simulink model "LPV_TorqueTracker_DT_CP_LMI_II_v3"  (R2018a)
settings: Solver=VariableStepAuto  StartTime=0  StopTime=FA.TMax  FixedStep=Simulation.DT  RelTol=1e-3  EnableMultiTasking=on
undefined symbols (not defined in the file or in its folder): Control, DiscIntNeverNeededParam, FA, OutList, Parameters, PitchControlParams, rpm2radps, strmatch, TorqueControlParams
libraries: simulink_extras x1
settings Model: ExtModeTrigMode=oneshot  ExtModeArmWhenConnect=off  Creator=Dana Martin  LastModifiedBy=dmartin
settings DataIOCC: SaveFormat=Array  SaveOutput=off  InspectSignalLogs=on  SignalLoggingName=sigsOut  OutputTimes=[0:500]/50
settings OptimizationCC: BooleanDataType=off  ExpressionDepthLimit=2147483647  InitFltsAndDblsToZero=on  LifeSpan=inf
settings DebuggingCC: SignalRangeChecking=warning  SaveWithParameterizedLinksMsg=none  UnderspecifiedInitializationDetection=Classic  MergeDetectMultiDrivingBlocksExec=none  SignalResolutionControl=TryResolveAllWithWarning  TimeAdjustmentMsg=warning  MultiTaskDSMMsg=warning  MultiTaskCondExecSysMsg=warning  ParameterUnderflowMsg=warning  UnderSpecifiedDataTypeMsg=warning  UnnecessaryDatatypeConvMsg=warning  VectorMatrixConversionMsg=warning  FcnCallInpInsideContextMsg=warning  SignalLabelMismatchMsg=warning  SFcnCompatibilityMsg=warning  UniqueDataStoreMsg=warning  AllowSymbolicDim=off  ModelReferenceIOMsg=warning  ModelReferenceVersionMismatchMessage=warning  ModelReferenceIOMismatchMessage=warning  StateNameClashWarn=warning  StrictBusMsg=WarnOnBusTreatedAsVector  NonBusSignalsTreatedAsBus=warning  SFUnexpectedBacktrackingDiag=warning  SFNoUnconditionalDefaultTransitionDiag=warning  SFExecutionAtInitializationDiag=none
settings HardwareCC: ProdBitPerPointer=32  ProdBitPerSizeT=32  ProdBitPerPtrDiffT=32  ProdLargestAtomicFloat=None  ProdIntDivRoundTo=Undefined  ProdEndianess=Unspecified  ProdWordSize=32  ProdHWDeviceType=32-bit Generic  TargetBitPerPointer=64  TargetBitPerSizeT=64  TargetBitPerPtrDiffT=64  TargetLongLongMode=on  TargetIntDivRoundTo=Zero  TargetEndianess=LittleEndian  TargetWordSize=64  TargetHWDeviceType=MATLAB Host  ProdEqTarget=off
settings ModelReferenceCC: PropagateSignalLabelsOutOfModel=off
settings CodeAppCC: StateflowObjectComments=on
settings GRTTargetCC: TargetFcnLib=ansi_tfl_tmw.mat  TargetLangStandard=C89/C90 (ANSI)  ModelReferenceCompliant=off  GeneratePreprocessorConditionals=Disable all  CombineOutputUpdateFcns=off  GRTInterface=on
settings ConfigComp: CovMetricSettings=dw  CovHtmlReporting=on  CovSaveCumulativeToWorkspaceVar=on  CovSaveSingleToWorkspaceVar=on  CovExternalEMLEnable=off  CovSFcnEnable=off

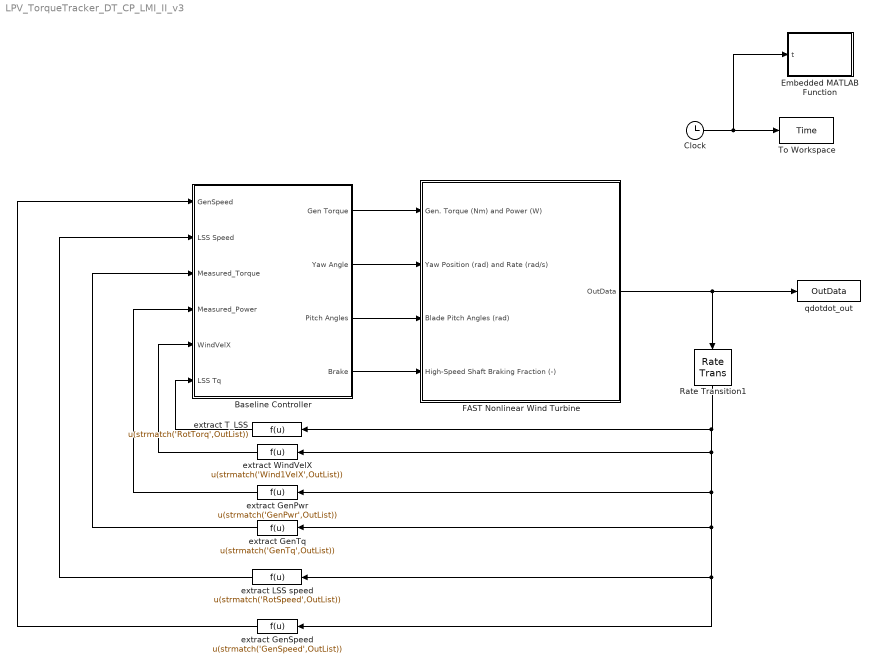
== system LPV_TorqueTracker_DT_CP_LMI_II_v3 ==
  Baseline Controller : Subsystem
  Clock : Clock
  Embedded MATLAB Function : MATLAB Function  TreatAsAtomicUnit=on
  FAST Nonlinear Wind Turbine : Subsystem  mask(FAST Nonlinear Wind Turbine){}
      mask help: This block contains the FAST S-Function.
      mask init:
      | clear FAST_SFunc
  Rate Transition1 : RateTransition
  To Workspace : ToWorkspace  VariableName=Time  SampleTime=FA.DT
  extract GenPwr : Fcn  Expr=u(strmatch('GenPwr',OutList))
  extract GenSpeed : Fcn  Expr=u(strmatch('GenSpeed',OutList))
  extract GenTq : Fcn  Expr=u(strmatch('GenTq',OutList))
  extract LSS speed : Fcn  Expr=u(strmatch('RotSpeed',OutList))
  extract T_LSS : Fcn  Expr=u(strmatch('RotTorq',OutList))
  extract WindVelX : Fcn  Expr=u(strmatch('Wind1VelX',OutList))
  qdotdot_out : ToWorkspace  VariableName=OutData  SaveFormat=Structure With Time  SampleTime=-1
  wires:
  Clock/1 -> Embedded MATLAB Function/1(t), To Workspace/1
  Baseline Controller/1(Gen Torque) -> FAST Nonlinear Wind Turbine/1(Gen. Torque (Nm) and Power (W))
  Baseline Controller/3(Pitch Angles) -> FAST Nonlinear Wind Turbine/3(Blade Pitch Angles (rad))
  extract GenSpeed/1 -> Baseline Controller/1(GenSpeed)
  Baseline Controller/2(Yaw Angle) -> FAST Nonlinear Wind Turbine/2(Yaw Position (rad) and Rate (rad/s))
  Baseline Controller/4(Brake) -> FAST Nonlinear Wind Turbine/4(High-Speed Shaft Braking Fraction (-))
  extract LSS speed/1 -> Baseline Controller/2(LSS Speed)
  extract GenPwr/1 -> Baseline Controller/4(Measured_Power)
  FAST Nonlinear Wind Turbine/1(OutData) -> qdotdot_out/1, Rate Transition1/1
  extract GenTq/1 -> Baseline Controller/3(Measured_Torque)
  extract WindVelX/1 -> Baseline Controller/5(WindVelX)
  extract T_LSS/1 -> Baseline Controller/6(LSS Tq)
  Rate Transition1/1 -> extract T_LSS/1, extract WindVelX/1, extract LSS speed/1, extract GenSpeed/1, extract GenTq/1, extract GenPwr/1

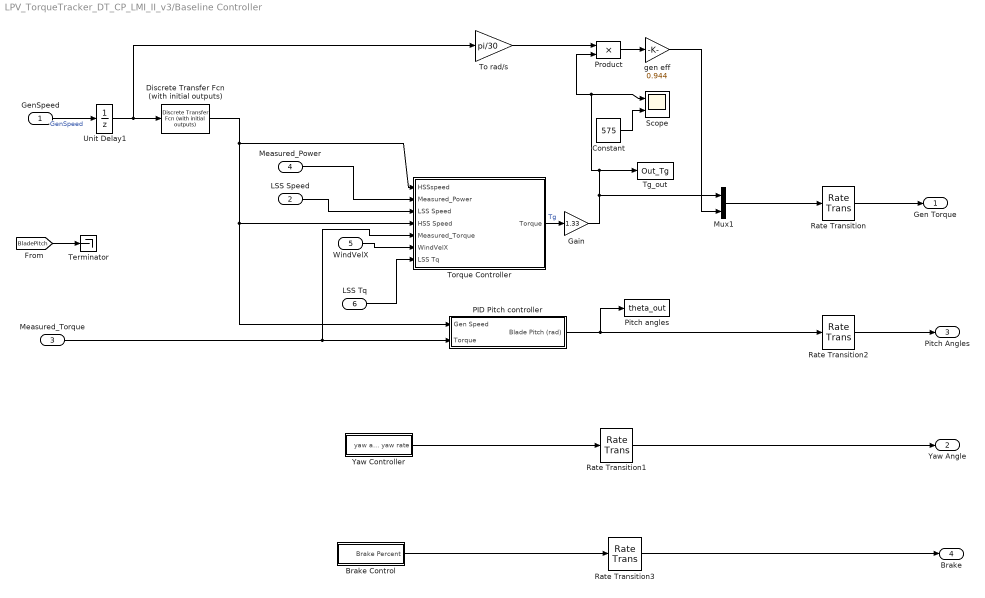
== system LPV_TorqueTracker_DT_CP_LMI_II_v3/Baseline Controller ==
  GenSpeed : Inport
  LSS Speed : Inport  Port=2
  Measured_Torque : Inport  Port=3
  Measured_Power : Inport  Port=4
  WindVelX : Inport  Port=5
  LSS Tq : Inport  Port=6
  Brake Control : Subsystem
  Constant : Constant  Value=575
  Discrete Transfer Fcn (with initial outputs) : simulink_extras/Additional Discrete/Discrete Transfer Fcn (with initial outputs)  N=Parameters.LPF.LPnum  D=Parameters.LPF.LPden  U0=Parameters.Turbine.IC.Wg  Y0=Parameters.Turbine.IC.Wg  TS=FA.DT
      settings: SourceProductName=Simulink  SourceProductBaseCode=SL
  Gain : Gain  Gain=1.33
  Mux1 : Mux  Inputs=2
  PID Pitch controller : Subsystem
      settings: MinAlgLoopOccurrences=on
  "Pitch angles " : ToWorkspace  VariableName=theta_out  SampleTime=FA.DT
  Product : Product  RndMeth=Zero
  Rate Transition : RateTransition  InitialCondition=Parameters.Turbine.IC.Tg
  Rate Transition1 : RateTransition
  Rate Transition2 : RateTransition  InitialCondition=Parameters.Turbine.IC.Bp
  Rate Transition3 : RateTransition
  Scope : Scope  NumInputPorts=2
  Terminator : Terminator
  Tg_out : ToWorkspace  VariableName=Out_Tg
      settings: MaxDataPoints=Inf
  To rad/s : Gain  Gain=pi/30
  Torque Controller : Subsystem
  Unit Delay1 : UnitDelay  InitialCondition=Parameters.Turbine.IC.Wg  SampleTime=FA.DT
  Yaw Controller : Subsystem
  gen eff : Gain  Gain=0.944
  Gen Torque : Outport
  Yaw Angle : Outport  Port=2
  Pitch Angles : Outport  Port=3
  Brake : Outport  Port=4
  wires:
  Mux1/1 -> Rate Transition/1
  Product/1 -> gen eff/1
  Discrete Transfer Fcn (with initial outputs)/1 -> Torque Controller/4(HSS Speed), PID Pitch controller/1(Gen Speed), Torque Controller/1(HSSspeed)
  Unit Delay1/1 -> Discrete Transfer Fcn (with initial outputs)/1, To rad/s/1
  PID Pitch controller/1(Blade Pitch (rad)) -> Rate Transition2/1, "Pitch angles "/1
  Rate Transition/1 -> Gen Torque/1
  Rate Transition2/1 -> Pitch Angles/1
  To rad/s/1 -> Product/1
  gen eff/1 -> Mux1/2
  GenSpeed/1 -> Unit Delay1/1  "GenSpeed"
  Torque Controller/1(Torque) -> Gain/1  "Tg"
  LSS Speed/1 -> Torque Controller/3(LSS Speed)
  Yaw Controller/1(yaw and yaw rate) -> Rate Transition1/1
  Brake Control/1(Brake Percent) -> Rate Transition3/1
  Rate Transition3/1 -> Brake/1
  Measured_Torque/1 -> PID Pitch controller/2(Torque), Torque Controller/5(Measured_Torque)
  Measured_Power/1 -> Torque Controller/2(Measured_Power)
  Rate Transition1/1 -> Yaw Angle/1
  WindVelX/1 -> Torque Controller/6(WindVelX)
  [BladePitch] -> Terminator/1
  LSS Tq/1 -> Torque Controller/7(LSS Tq)
  Gain/1 -> Product/2, Scope/1, Tg_out/1, Mux1/1
  Constant/1 -> Scope/2

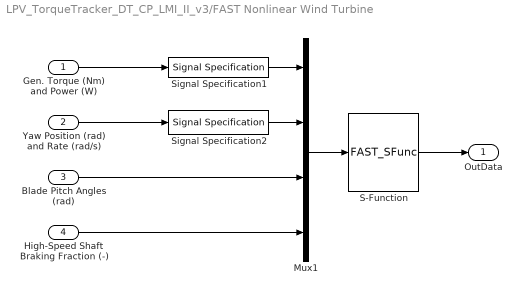
== system LPV_TorqueTracker_DT_CP_LMI_II_v3/FAST Nonlinear Wind Turbine ==
  Gen. Torque (Nm) and Power (W) : Inport
  Yaw Position (rad) and Rate (rad/s) : Inport  Port=2
  Blade Pitch Angles (rad) : Inport  Port=3
  High-Speed Shaft Braking Fraction (-) : Inport  Port=4
  Mux1 : Mux
  S-Function : S-Function  FunctionName=FAST_SFunc  Parameters=FAST_InputFileName, FA.TMax, 0  SFunctionDeploymentMode=off  EnableBusSupport=off
  Signal Specification1 : SignalSpecification  OutDataTypeStr=double  Dimensions=2
  Signal Specification2 : SignalSpecification  OutDataTypeStr=double  Dimensions=2
  OutData : Outport
  wires:
  Gen. Torque (Nm) and Power (W)/1 -> Signal Specification1/1
  S-Function/1 -> OutData/1
  Mux1/1 -> S-Function/1
  Blade Pitch Angles (rad)/1 -> Mux1/3
  Yaw Position (rad) and Rate (rad/s)/1 -> Signal Specification2/1
  Signal Specification1/1 -> Mux1/1
  Signal Specification2/1 -> Mux1/2
  High-Speed Shaft Braking Fraction (-)/1 -> Mux1/4

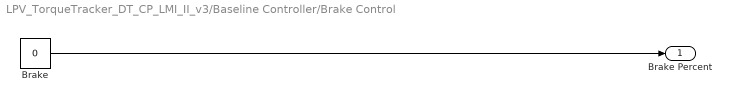
== system LPV_TorqueTracker_DT_CP_LMI_II_v3/Baseline Controller/Brake Control ==
  Brake : Constant  Value=0  SampleTime=-1
  Brake Percent : Outport
  wires:
  Brake/1 -> Brake Percent/1

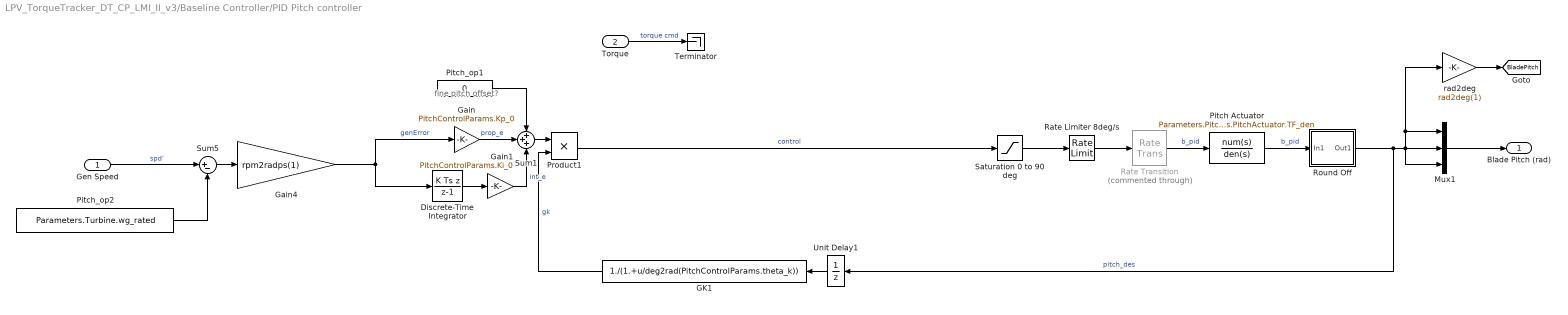
== system LPV_TorqueTracker_DT_CP_LMI_II_v3/Baseline Controller/PID Pitch controller ==
  note: fine pitch offset?
  Gen Speed : Inport
  Torque : Inport  Port=2
  Discrete-Time Integrator : DiscreteIntegrator  IntegratorMethod=Integration: Backward Euler  gainval=1  InitialCondition=deg2rad(Parameters.Turbine.fine_pitch)/(PitchControlParams.Ki_0)/(1./(1.+deg2rad(Parameters.Turbine.fine_pitch)/PitchControlParams.theta_k))  SampleTime=Control.DT  LimitOutput=on  UpperSaturationLimit=5*1.570796/(PitchControlParams.Ki_0)/(1./(1.+1.570796/PitchControlParams.theta_k))  LowerSaturationLimit=deg2rad(Parameters.Turbine.fine_pitch)/(PitchControlParams.Ki_0)/(1./(1.+deg2rad(Parameters.Turbine.fine_pitch)/PitchControlParams.theta_k))  ICPrevOutput=DiscIntNeverNeededParam  ICPrevScaledInput=DiscIntNeverNeededParam
  GK1 : Fcn  Expr=1./(1.+u/deg2rad(PitchControlParams.theta_k))
  Gain : Gain  Gain=PitchControlParams.Kp_0
  Gain1 : Gain  Gain=PitchControlParams.Ki_0
  Gain4 : Gain  Gain=rpm2radps(1)
  Mux1 : Mux  Inputs=3
  Pitch Actuator : TransferFcn  Numerator=Parameters.PitchActuator.TF_num  Denominator=Parameters.PitchActuator.TF_den
  Pitch_op1 : Constant  Value=0  SampleTime=Control.DT
  Pitch_op2 : Constant  Value=Parameters.Turbine.wg_rated  SampleTime=Control.DT
  Product1 : Product  RndMeth=Zero
  Rate Limiter 8deg/s : RateLimiter  RisingSlewLimit=8*pi/180  FallingSlewLimit=-8*pi/180  SampleTimeMode=inherited  InitialCondition=deg2rad(0)
  Rate Transition : RateTransition  Commented=through
  Round Off : Subsystem
  Saturation 0 to 90 deg : Saturate  UpperLimit=90*pi/180  LowerLimit=deg2rad(Parameters.Turbine.fine_pitch)
  Sum1 : Sum  Inputs=+++
  Sum5 : Sum  Inputs=|+-  SaturateOnIntegerOverflow=on  InputSameDT=on  OutDataTypeStr=Inherit: Same as first input
  Terminator : Terminator
  Unit Delay1 : UnitDelay  InitialCondition=Parameters.Turbine.IC.Wg  SampleTime=Control.DT
  rad2deg : Gain  Gain=rad2deg(1)
  Blade Pitch (rad) : Outport
  tag scope: BladePitch=global
  wires:
  Pitch_op2/1 -> Sum5/2
  Gen Speed/1 -> Sum5/1  "spd'"
  Discrete-Time Integrator/1 -> Gain1/1
  Gain/1 -> Sum1/2  "prop_e"
  Pitch_op1/1 -> Sum1/1
  Gain1/1 -> Sum1/3  "int_e"
  Sum1/1 -> Product1/1
  Unit Delay1/1 -> GK1/1
  Saturation 0 to 90 deg/1 -> Rate Limiter 8deg/s/1
  GK1/1 -> Product1/2  "gk"
  Rate Transition/1 -> Pitch Actuator/1  "b_pid"
  Rate Limiter 8deg/s/1 -> Rate Transition/1
  Sum5/1 -> Gain4/1
  Round Off/1(Out1) -> Mux1/3, rad2deg/1, Mux1/1, Mux1/2, Unit Delay1/1  "pitch_des"
  Torque/1 -> Terminator/1  "torque cmd"
  Product1/1 -> Saturation 0 to 90 deg/1  "control"
  Gain4/1 -> Discrete-Time Integrator/1, Gain/1  "genError"
  Mux1/1 -> Blade Pitch (rad)/1
  rad2deg/1 -> [BladePitch]
  Pitch Actuator/1 -> Round Off/1(In1)  "b_pid"

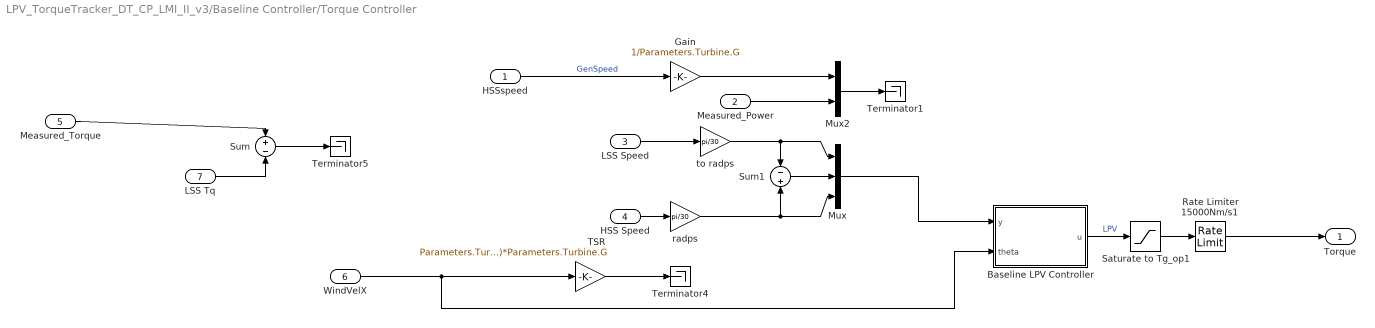
== system LPV_TorqueTracker_DT_CP_LMI_II_v3/Baseline Controller/Torque Controller ==
  HSSspeed : Inport
  Measured_Power : Inport  Port=2
  LSS Speed : Inport  Port=3
  HSS Speed : Inport  Port=4
  Measured_Torque : Inport  Port=5
  WindVelX : Inport  Port=6
  LSS Tq : Inport  Port=7
  Baseline LPV Controller : Subsystem  TreatAsAtomicUnit=on
      settings: MinAlgLoopOccurrences=on
  Gain : Gain  Gain=1/Parameters.Turbine.G
  Mux : Mux  Inputs=3
  Mux2 : Mux  Inputs=2
  Rate Limiter 15000Nm/s1 : RateLimiter  RisingSlewLimit=15000  FallingSlewLimit=-15000  SampleTimeMode=inherited  InitialCondition=Parameters.Turbine.IC.Tg
  Saturate to Tg_op1 : Saturate  UpperLimit=TorqueControlParams.T_rated  LowerLimit=0
  Sum : Sum  Inputs=+-
  Sum1 : Sum  Inputs=-+
  TSR : Gain  Gain=Parameters.Turbine.la_max/Parameters.Turbine.R*(30/pi)*Parameters.Turbine.G
  Terminator1 : Terminator
  Terminator4 : Terminator
  Terminator5 : Terminator
  radps : Gain  Gain=pi/30
  to radps : Gain  Gain=pi/30
  Torque : Outport
  wires:
  Measured_Torque/1 -> Sum/1
  Baseline LPV Controller/1(u) -> Saturate to Tg_op1/1  "LPV"
  HSSspeed/1 -> Gain/1  "GenSpeed"
  WindVelX/1 -> Baseline LPV Controller/2(theta), TSR/1
  TSR/1 -> Terminator4/1
  Measured_Power/1 -> Mux2/2
  LSS Tq/1 -> Sum/2
  Gain/1 -> Mux2/1
  HSS Speed/1 -> radps/1
  radps/1 -> Sum1/2, Mux/3
  Mux2/1 -> Terminator1/1
  Sum/1 -> Terminator5/1
  Sum1/1 -> Mux/2
  LSS Speed/1 -> to radps/1
  to radps/1 -> Sum1/1, Mux/1
  Saturate to Tg_op1/1 -> Rate Limiter 15000Nm/s1/1
  Rate Limiter 15000Nm/s1/1 -> Torque/1
  Mux/1 -> Baseline LPV Controller/1(y)

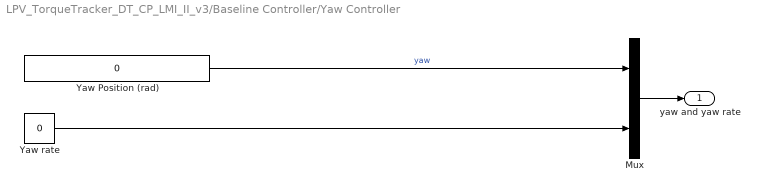
== system LPV_TorqueTracker_DT_CP_LMI_II_v3/Baseline Controller/Yaw Controller ==
  Mux : Mux  Inputs=2
  Yaw Position (rad) : Constant  Value=0  SampleTime=-1
  Yaw rate : Constant  Value=0  SampleTime=-1
  yaw and yaw rate : Outport
  wires:
  Mux/1 -> yaw and yaw rate/1
  Yaw Position (rad)/1 -> Mux/1  "yaw"
  Yaw rate/1 -> Mux/2

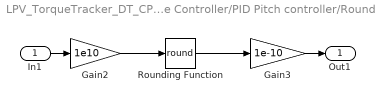
== system LPV_TorqueTracker_DT_CP_LMI_II_v3/Baseline Controller/PID Pitch controller/Round Off ==
  In1 : Inport
  Gain2 : Gain  Gain=1e10
  Gain3 : Gain  Gain=1e-10
  Rounding Function : Rounding  Operator=round
  Out1 : Outport
  wires:
  Gain2/1 -> Rounding Function/1
  Rounding Function/1 -> Gain3/1
  Gain3/1 -> Out1/1
  In1/1 -> Gain2/1

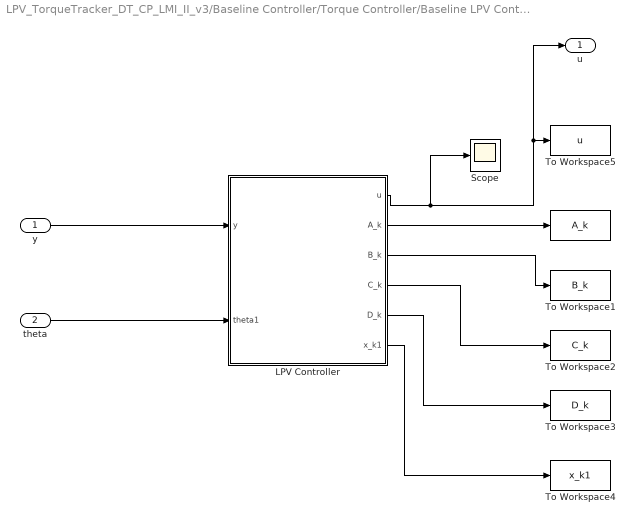
== system LPV_TorqueTracker_DT_CP_LMI_II_v3/Baseline Controller/Torque Controller/Baseline LPV Controller ==
  y : Inport
  theta : Inport  Port=2
  " " : ToWorkspace  VariableName=A_k  SaveFormat=Structure With Time  SampleTime=-1
      settings: Decimation=3
  LPV Controller : MATLAB Function  TreatAsAtomicUnit=on
      settings: MinAlgLoopOccurrences=on
  Scope : Scope
  To Workspace1 : ToWorkspace  VariableName=B_k  SaveFormat=Structure With Time  SampleTime=-1
      settings: Decimation=3
  To Workspace2 : ToWorkspace  VariableName=C_k  SaveFormat=Structure With Time  SampleTime=-1
      settings: Decimation=3
  To Workspace3 : ToWorkspace  VariableName=D_k  SaveFormat=Structure With Time  SampleTime=-1
      settings: Decimation=3
  To Workspace4 : ToWorkspace  VariableName=x_k1  SaveFormat=Structure With Time  SampleTime=-1
      settings: Decimation=3
  To Workspace5 : ToWorkspace  VariableName=u  SaveFormat=Structure With Time  SampleTime=-1
      settings: Decimation=3
  u : Outport
  wires:
  theta/1 -> LPV Controller/2(theta1)
  y/1 -> LPV Controller/1(y)
  LPV Controller/1(u) -> Scope/1, u/1, To Workspace5/1
  LPV Controller/3(B_k) -> To Workspace1/1
  LPV Controller/2(A_k) -> " "/1
  LPV Controller/4(C_k) -> To Workspace2/1
  LPV Controller/5(D_k) -> To Workspace3/1
  LPV Controller/6(x_k1) -> To Workspace4/1

== matlab function LPV_TorqueTracker_DT_CP_LMI_II_v3/Baseline Controller/Torque Controller/Baseline LPV Controller/LPV Controller ==
  data: y input; theta1 input; u output; A_k output; B_k output; C_k output; D_k output; x_k1 output
function [u,  A_k, B_k, C_k, D_k, x_k1]   = LPVController(y, theta1)
persistent x_k;

if isempty(x_k)
    x_k = zeros(3,1); 
end

K_bar =[ 2.8575e-52*theta1 + 2.2697e-19,    1.4302e-68*theta1 + 1.6078e-25,    8.0867e-69*theta1 + 5.2536e-26, -2.2214e-19;
  - 1.5363e-29*theta1 - 10180.0, - 7.6897e-46*theta1 - 0.000088866, - 4.3479e-46*theta1 - 0.000058681,     10232.0;
    9.4742e-30*theta1 + 10806.0,       4.742e-46*theta1 + 0.019193,      2.6812e-46*theta1 + 0.006221,    -10140.0;
                        -622.75,                           0.04227,                          0.022752,     -12.264];

A_k        = K_bar(1:3,1:3);
Controller.A_k = A_k;

B_k        = K_bar(1:3,4);
Controller.B_k = B_k;

C_k        = K_bar(4,1:3);
Controller.C_k = C_k;

D_k        = K_bar(4,4);
Controller.B_k = D_k;

x_k1       = A_k*x_k+B_k*y(1);
Controller.x_k1 = x_k1;

u          = C_k*x_k+D_k*y(1); 

x_k        = x_k1;

end

== matlab function LPV_TorqueTracker_DT_CP_LMI_II_v3/Embedded MATLAB Function ==
  data: t input
function TellTime(t)

if t==0
    Tsim=t
elseif rem(t,50)==0
    Tsim=t
end
